simulink library "lib_joint_impctrl"  (Simulink 8.5)
settings: Solver=ode45  StartTime=0.0  StopTime=10.0  RelTol=1e-3
undefined symbols (not defined in the file): atlas_arm_lr, B, D, K_d, K_ext_c, K_ext_o, K_fri_o, K_O, K_obs_c, K_qD_d, K_qDD_d, K_tau_a, K_tau_c, K_tau_D, K_tau_e, K_tau_f, K_tau_g, K_tau_K, K_tau_o, MPV_arm_damp, MPV_arm_model, qD_th, T, T1, tau_c, tau_th
libraries: lib_joint_impctrl x7, atlas_dynamic_library x4
settings Model: Creator=knoechelmann  LastModifiedBy=prothese  CovSFcnEnable=off

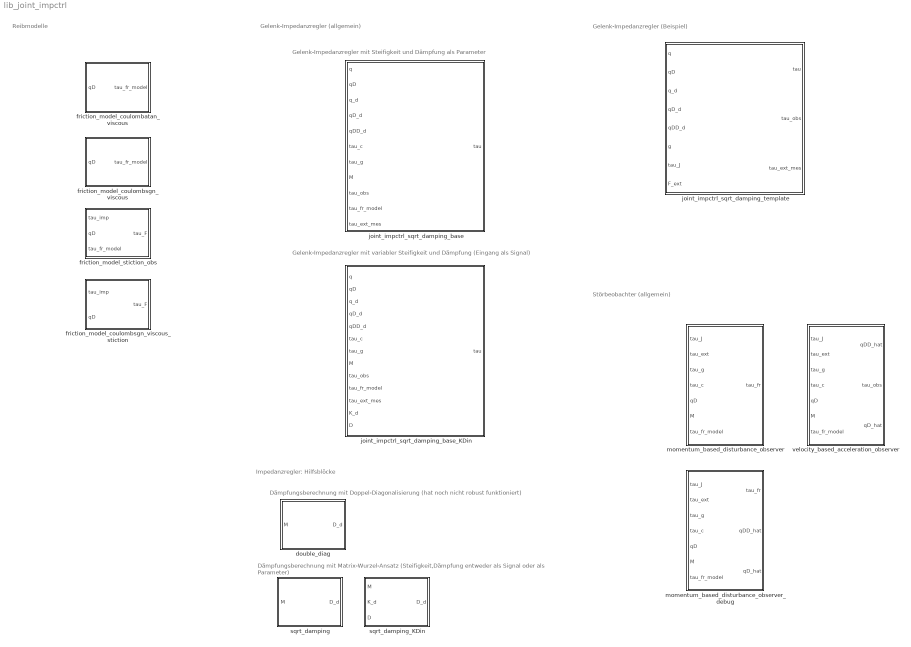
== system lib_joint_impctrl ==
  note: Dämpfungsberechnung mit Doppel-Diagonalisierung (hat noch nicht robust funktioniert)
  note: Dämpfungsberechnung mit Matrix-Wurzel-Ansatz (Steifigkeit,Dämpfung entweder als Signal oder als Parameter)
  note: Gelenk-Impedanzregler mit Steifigkeit und Dämpfung als Parameter
  note: Gelenk-Impedanzregler mit variabler Steifigkeit und Dämpfung (Eingang als Signal)
  note: Gelenk-Impedanzregler (Beispiel)
  note: Störbeobachter (allgemein)
  note: Gelenk-Impedanzregler (allgemein)
  note: Impedanzregler: Hilfsblöcke
  note: Reibmodelle
  double_diag : Subsystem  TreatAsAtomicUnit=on  mask{K_d=K_d, D=D}
  friction_model_coulombatan_viscous : Subsystem  TreatAsAtomicUnit=on  mask{tau_c=tau_c, B=B}
      mask prompts: tau_c "tau_c (vector with coulomb friction momentums for all joints)"; B "B (vector with viscous friction coefficients of all joints)"
  friction_model_coulombsgn_viscous : Subsystem  TreatAsAtomicUnit=on  mask{tau_c=tau_c, B=B}
      mask prompts: tau_c "tau_c (vector with coulomb friction momentums for all joints)"; B "B (vector with viscous friction coefficients of all joints)"
  friction_model_coulombsgn_viscous_stiction : Subsystem  TreatAsAtomicUnit=on  mask{tau_c=tau_c, B=B, qD_th=qD_th, tau_th=tau_th}
      mask prompts: tau_c "tau_c (vector with coulomb friction momentums for all joints)"; B "B (vector with viscous friction coefficients of all joints)"; qD_th "qD_th (vector with theshold velocities for stiction)"; tau_th "tau_th (vector with kick-in momentums for stiction compensation)"
  friction_model_stiction_obs : Subsystem  TreatAsAtomicUnit=on  mask{tau_c=tau_c, B=B, qD_th=qD_th, tau_th=tau_th}
      mask prompts: tau_c "tau_c (vector with coulomb friction momentums for all joints)"; B "B (vector with viscous friction coefficients of all joints)"; qD_th "qD_th (vector with theshold velocities for stiction)"; tau_th "tau_th (vector with kick-in momentums for stiction compensation)"
  joint_impctrl_sqrt_damping_base : Subsystem  TreatAsAtomicUnit=on  mask(Joint Impedance Controller Base){K_d=K_d, D=D, K_tau_g=K_tau_g, K_tau_c=K_tau_c, K_tau_K=K_tau_K, K_tau_D=K_tau_D, K_tau_a=K_tau_a, K_tau_f=K_tau_f, K_tau_e=K_tau_e, K_tau_o=K_tau_o, K_qD_d=K_qD_d, K_qDD_d=K_qDD_d, K_ext_c=K_ext_c, K_obs_c=K_obs_c, tau_c=tau_c, B=B, qD_th=qD_th, tau_th=tau_th}
      mask prompts: K_d "K_d (desired stiffness)"; D "D (diagonal matrix with desired damping coefficients)"; K_tau_g "K_tau_g (gain of gravity compensation)"; K_tau_c "K_tau_c (gain of corriolis- and inertia compensation)"; K_tau_K "K_tau_K (gain of stiffness component)"; K_tau_D "K_tau_D (gain of damping component)"; K_tau_a "K_tau_a (gain of acceleration component)"; K_tau_f "K_tau_f (gain of model based friction compensation)"; K_tau_e "K_tau_e (gain of compensation of external torque measurd via hand sensor)"; K_tau_o "K_tau_o (gain of compensation of disturbance observer torques)"; K_qD_d "K_qD_d (gain of desired velocity)"; K_qDD_d "K_qDD_d (gain of desired acceleration)"; K_ext_c "K_ext_c (input gain to deside, wether to trigger friction compensation via the measured external torque)"; K_obs_c "K_obs_c (input gain to deside, wether to trigger friction compensation via the observed torque)"; tau_c "tau_c (vector with coulomb friction momentums for all joints)"; B "B (vector with viscous friction coefficients of all joints)"; qD_th "qD_th (vector with theshold velocities for stiction)"; tau_th "tau_th (vector with kick-in momentums for stiction compensation)"
      mask help:
      | Hardware independent impedance controller base block with matrix
      | squareroot damping design. For a better testing, all partial mo-
      | mentums can be individually scaled. Coulomb-, viscous friction
      | and Stribeck stiction is taken into account for friction compen-
      | sation.
  joint_impctrl_sqrt_damping_base_KDin : Subsystem  TreatAsAtomicUnit=on  mask(Joint Impedance Controller Base){K_tau_g=K_tau_g, K_tau_c=K_tau_c, K_tau_K=K_tau_K, K_tau_D=K_tau_D, K_tau_a=K_tau_a, K_tau_f=K_tau_f, K_tau_e=K_tau_e, K_tau_o=K_tau_o, K_qD_d=K_qD_d, K_qDD_d=K_qDD_d, K_ext_c=K_ext_c, K_obs_c=K_obs_c, tau_c=tau_c, B=B, qD_th=qD_th, tau_th=tau_th}
      mask prompts: K_tau_g "K_tau_g (gain of gravity compensation)"; K_tau_c "K_tau_c (gain of corriolis- and inertia compensation)"; K_tau_K "K_tau_K (gain of stiffness component)"; K_tau_D "K_tau_D (gain of damping component)"; K_tau_a "K_tau_a (gain of acceleration component)"; K_tau_f "K_tau_f (gain of model based friction compensation)"; K_tau_e "K_tau_e (gain of compensation of external torque measurd via hand sensor)"; K_tau_o "K_tau_o (gain of compensation of disturbance observer torques)"; K_qD_d "K_qD_d (gain of desired velocity)"; K_qDD_d "K_qDD_d (gain of desired acceleration)"; K_ext_c "K_ext_c (input gain to deside, wether to trigger friction compensation via the measured external torque)"; K_obs_c "K_obs_c (input gain to deside, wether to trigger friction compensation via the observed torque)"; tau_c "tau_c (vector with coulomb friction momentums for all joints)"; B "B (vector with viscous friction coefficients of all joints)"; qD_th "qD_th (vector with theshold velocities for stiction)"; tau_th "tau_th (vector with kick-in momentums for stiction compensation)"
      mask help:
      | Hardware independent impedance controller base block with matrix
      | squareroot damping design. For a better testing, all partial mo-
      | mentums can be individually scaled. Coulomb-, viscous friction
      | and Stribeck stiction is taken into account for friction compen-
      | sation.
  joint_impctrl_sqrt_damping_template : Subsystem  TreatAsAtomicUnit=on  SystemSampleTime=T  mask(Atlas Joint Impedance Controller){K_d=K_d, D=D, K_tau_g=K_tau_g, K_tau_c=K_tau_c, K_tau_K=K_tau_K, K_tau_D=K_tau_D, K_tau_a=K_tau_a, K_tau_f=K_tau_f, K_tau_e=K_tau_e, K_tau_o=K_tau_o, K_qD_d=K_qD_d, K_qDD_d=K_qDD_d, K_ext_c=K_ext_c, K_obs_c=K_obs_c, K_fri_o=K_fri_o, K_ext_o=K_ext_o, MPV_arm_damp=MPV_arm_damp, MPV_arm_model=MPV_arm_model, tau_c=tau_c, B=B, qD_th=qD_th, tau_th=tau_th, K_O=K_O, T=T, atlas_arm_lr=atlas_arm_lr, T1=T1}
      mask prompts: K_d "K_d (desired stiffness)"; D "D (diagonal matrix with desired damping coefficients)"; K_tau_g "K_tau_g (gain of gravity compensation)"; K_tau_c "K_tau_c (gain of corriolis- and inertia compensation)"; K_tau_K "K_tau_K (gain of stiffness component)"; K_tau_D "K_tau_D (gain of damping component)"; K_tau_a "K_tau_a (gain of acceleration component)"; K_tau_f "K_tau_f (gain of model based friction compensation)"; K_tau_e "K_tau_e (gain of compensation of external torque measurd via hand sensor)"; K_tau_o "K_tau_o (gain of compensation of disturbance observer torques)"; K_qD_d "K_qD_d (gain of desired velocity)"; K_qDD_d "K_qDD_d (gain of desired acceleration)"; K_ext_c "K_ext_c (input gain to deside, wether to trigger friction compensation via the measured external torque)"; K_obs_c "K_obs_c (input gain to deside, wether to trigger friction compensation via the observed torque)"; K_fri_o "K_fri_o (input gain of friction model torques for observer)"; K_ext_o "K_ext_o (input gain of external torque for observer)"; MPV_arm_damp "MPV_damp (base parameter vector for damping calculation)"; MPV_arm_model "MPV_model (base parameter vector for dynamic model calculation)"; tau_c "tau_c (vector with coulomb friction momentums for all joints)"; B "B (vector with viscous friction coefficients of all joints)"; qD_th "qD_th (vector with theshold velocities for stiction)"; tau_th "tau_th (vector with kick-in momentums for stiction compensation)"; K_O "K_O (friction observer gain)"; T "T (sample time (important for friction observer))"; atlas_arm_lr "atlas_arm_lr (flag for left or right side)"; T1 "T1 (low pass filter time constant for inertia matrix)"
      mask help:
      | Hardware dependent full impedance controller block with matrix
      | squareroot damping design for the atlas robot. For a better
      | testing, all partial momentums can be individually scaled.
      | Coulomb-, viscous friction and Stribeck stiction is taken into
      | account for friction compensation.
  momentum_based_disturbance_observer : Subsystem  TreatAsAtomicUnit=on  SystemSampleTime=T  mask{K_O=K_O, T=T, T1=T1, tau_out_max=30*ones(6,1)}
      mask prompts: K_O "K_O (Observer gain)"; T "T (sampletime)"; T1 "T1 (low pass differentiator time constant)"; tau_out_max "tau_out_max (safety limit for output, output will be limited to lie in between -tau_out_max and tau_out_max)"
  momentum_based_disturbance_observer_debug : Subsystem  TreatAsAtomicUnit=on  SystemSampleTime=T  mask{K_O=K_O, T=T, T1=T1, tau_out_max=30*ones(6,1)}
      mask prompts: K_O "K_O (Observer gain)"; T "T (sampletime)"; T1 "T1 (low pass differentiator time constant)"; tau_out_max "tau_out_max (safety limit for output, output will be limited to lie in between -tau_out_max and tau_out_max)"
  sqrt_damping : Subsystem  TreatAsAtomicUnit=on  mask{K_d=K_d, D=D}
  sqrt_damping_KDin : Subsystem  TreatAsAtomicUnit=on
  velocity_based_acceleration_observer : Subsystem  TreatAsAtomicUnit=on  SystemSampleTime=T  mask{K_O=K_O, T=T}
      mask prompts: K_O "K_O (Observer gain)"; T "T (sampletime)"

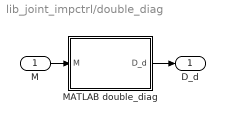
== system lib_joint_impctrl/double_diag ==
  M : Inport
  MATLAB double_diag : MATLAB Function  TreatAsAtomicUnit=on
  D_d : Outport
  wires:
  M/1 -> MATLAB double_diag/1(M)
  MATLAB double_diag/1(D_d) -> D_d/1

== system lib_joint_impctrl/friction_model_coulombatan_viscous ==
  qD : Inport
  atlas_friction_model_atan : MATLAB Function  TreatAsAtomicUnit=on
  tau_fr_model : Outport
  wires:
  qD/1 -> atlas_friction_model_atan/1(qD)
  atlas_friction_model_atan/1(tau_fr_model) -> tau_fr_model/1

== system lib_joint_impctrl/friction_model_coulombsgn_viscous ==
  qD : Inport
  atlas_friction_model : MATLAB Function  TreatAsAtomicUnit=on
  tau_fr_model : Outport
  wires:
  qD/1 -> atlas_friction_model/1(qD)
  atlas_friction_model/1(tau_fr_model) -> tau_fr_model/1

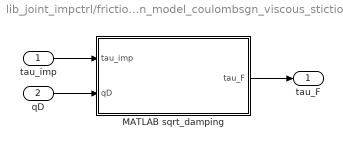
== system lib_joint_impctrl/friction_model_coulombsgn_viscous_stiction ==
  tau_imp : Inport
  qD : Inport  Port=2
  MATLAB sqrt_damping : MATLAB Function  TreatAsAtomicUnit=on
  tau_F : Outport
  wires:
  qD/1 -> MATLAB sqrt_damping/2(qD)
  MATLAB sqrt_damping/1(tau_F) -> tau_F/1
  tau_imp/1 -> MATLAB sqrt_damping/1(tau_imp)

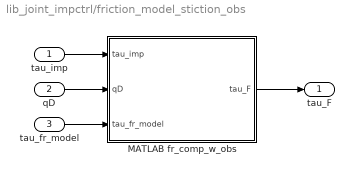
== system lib_joint_impctrl/friction_model_stiction_obs ==
  tau_imp : Inport
  qD : Inport  Port=2
  tau_fr_model : Inport  Port=3
  MATLAB fr_comp_w_obs : MATLAB Function  TreatAsAtomicUnit=on
  tau_F : Outport
  wires:
  qD/1 -> MATLAB fr_comp_w_obs/2(qD)
  MATLAB fr_comp_w_obs/1(tau_F) -> tau_F/1
  tau_imp/1 -> MATLAB fr_comp_w_obs/1(tau_imp)
  tau_fr_model/1 -> MATLAB fr_comp_w_obs/3(tau_fr_model)

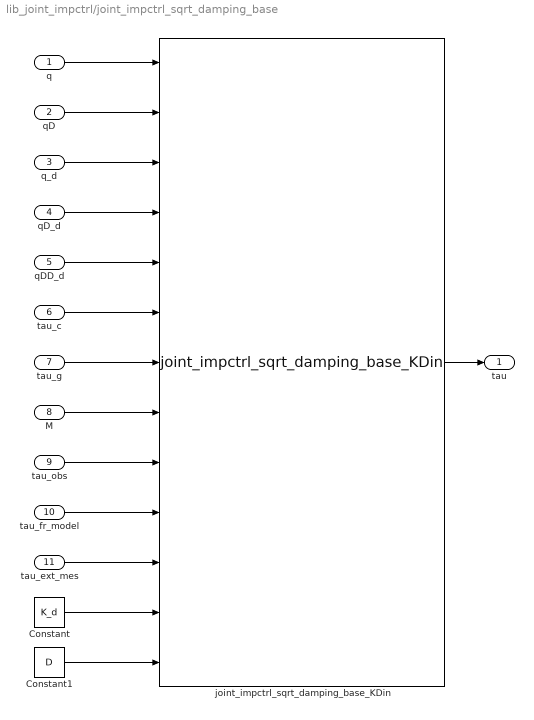
== system lib_joint_impctrl/joint_impctrl_sqrt_damping_base ==
  q : Inport
  qD : Inport  Port=2
  q_d : Inport  Port=3
  qD_d : Inport  Port=4
  qDD_d : Inport  Port=5
  tau_c : Inport  Port=6
  tau_g : Inport  Port=7
  M : Inport  Port=8
  tau_obs : Inport  Port=9
  tau_fr_model : Inport  Port=10
  tau_ext_mes : Inport  Port=11
  Constant : Constant  Value=K_d
  Constant1 : Constant  Value=D
  joint_impctrl_sqrt_damping_base_KDin : lib_joint_impctrl/joint_impctrl_sqrt_damping_base_KDin  K_tau_g=K_tau_g  K_tau_c=K_tau_c  K_tau_K=K_tau_K  K_tau_D=K_tau_D  K_tau_a=K_tau_a  K_tau_f=K_tau_f  K_tau_e=K_tau_e  K_tau_o=K_tau_o  K_qD_d=K_qD_d  K_qDD_d=K_qDD_d  K_ext_c=K_ext_c  K_obs_c=K_obs_c  tau_c=tau_c  B=B  qD_th=qD_th  tau_th=tau_th
  tau : Outport
  wires:
  joint_impctrl_sqrt_damping_base_KDin/1 -> tau/1
  tau_fr_model/1 -> joint_impctrl_sqrt_damping_base_KDin/10
  q/1 -> joint_impctrl_sqrt_damping_base_KDin/1
  q_d/1 -> joint_impctrl_sqrt_damping_base_KDin/3
  qD/1 -> joint_impctrl_sqrt_damping_base_KDin/2
  qD_d/1 -> joint_impctrl_sqrt_damping_base_KDin/4
  qDD_d/1 -> joint_impctrl_sqrt_damping_base_KDin/5
  tau_c/1 -> joint_impctrl_sqrt_damping_base_KDin/6
  tau_g/1 -> joint_impctrl_sqrt_damping_base_KDin/7
  tau_obs/1 -> joint_impctrl_sqrt_damping_base_KDin/9
  tau_ext_mes/1 -> joint_impctrl_sqrt_damping_base_KDin/11
  M/1 -> joint_impctrl_sqrt_damping_base_KDin/8
  Constant/1 -> joint_impctrl_sqrt_damping_base_KDin/12
  Constant1/1 -> joint_impctrl_sqrt_damping_base_KDin/13

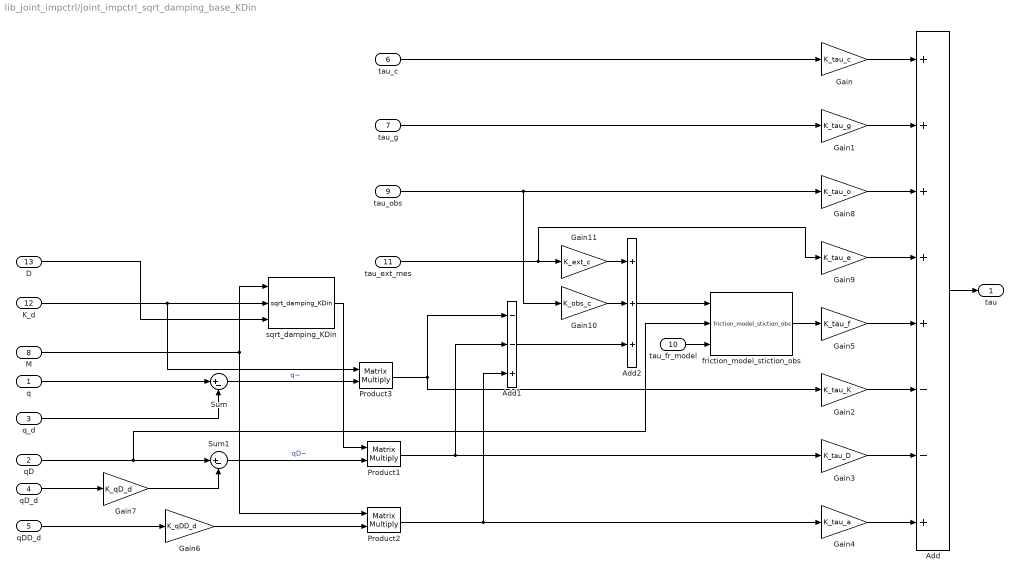
== system lib_joint_impctrl/joint_impctrl_sqrt_damping_base_KDin ==
  q : Inport
  qD : Inport  Port=2
  q_d : Inport  Port=3
  qD_d : Inport  Port=4
  qDD_d : Inport  Port=5
  tau_c : Inport  Port=6
  tau_g : Inport  Port=7
  M : Inport  Port=8
  tau_obs : Inport  Port=9
  tau_fr_model : Inport  Port=10
  tau_ext_mes : Inport  Port=11
  K_d : Inport  Port=12
  D : Inport  Port=13
  Add : Sum  Inputs=+++++--+
  Add1 : Sum  Inputs=--+
  Add2 : Sum  Inputs=+++
  Gain : Gain  Gain=K_tau_c
  Gain1 : Gain  Gain=K_tau_g
  Gain10 : Gain  Gain=K_obs_c
  Gain11 : Gain  Gain=K_ext_c
  Gain2 : Gain  Gain=K_tau_K
  Gain3 : Gain  Gain=K_tau_D
  Gain4 : Gain  Gain=K_tau_a
  Gain5 : Gain  Gain=K_tau_f
  Gain6 : Gain  Gain=K_qDD_d
  Gain7 : Gain  Gain=K_qD_d
  Gain8 : Gain  Gain=K_tau_o
  Gain9 : Gain  Gain=K_tau_e
  Product1 : Product  Multiplication=Matrix(*)
  Product2 : Product  Multiplication=Matrix(*)
  Product3 : Product  Multiplication=Matrix(*)
  Sum : Sum  Inputs=|+-
  Sum1 : Sum  Inputs=|+-
  friction_model_stiction_obs : lib_joint_impctrl/friction_model_stiction_obs  tau_c=tau_c  B=B  qD_th=qD_th  tau_th=tau_th
  sqrt_damping_KDin : lib_joint_impctrl/sqrt_damping_KDin  K_d=K_d  D=D
  tau : Outport
  wires:
  Gain6/1 -> Product2/2
  Gain7/1 -> Sum1/2
  q_d/1 -> Sum/2
  M/1 -> Product2/1, sqrt_damping_KDin/1
  q/1 -> Sum/1
  qD/1 -> friction_model_stiction_obs/2, Sum1/1
  qD_d/1 -> Gain7/1
  Sum1/1 -> Product1/2  "qD~"
  Sum/1 -> Product3/2  "q~"
  qDD_d/1 -> Gain6/1
  sqrt_damping_KDin/1 -> Product1/1
  Add/1 -> tau/1
  Product3/1 -> Gain2/1, Add1/1
  tau_g/1 -> Gain1/1
  tau_c/1 -> Gain/1
  Product1/1 -> Gain3/1, Add1/2
  Product2/1 -> Gain4/1, Add1/3
  Gain/1 -> Add/1
  Gain1/1 -> Add/2
  tau_obs/1 -> Gain8/1, Gain10/1
  tau_fr_model/1 -> friction_model_stiction_obs/3
  Gain5/1 -> Add/5
  Gain2/1 -> Add/6
  Gain3/1 -> Add/7
  Gain4/1 -> Add/8
  Gain8/1 -> Add/3
  tau_ext_mes/1 -> Gain9/1, Gain11/1
  Gain9/1 -> Add/4
  Add2/1 -> friction_model_stiction_obs/1
  Add1/1 -> Add2/3
  Gain10/1 -> Add2/2
  Gain11/1 -> Add2/1
  friction_model_stiction_obs/1 -> Gain5/1
  K_d/1 -> Product3/1, sqrt_damping_KDin/2
  D/1 -> sqrt_damping_KDin/3

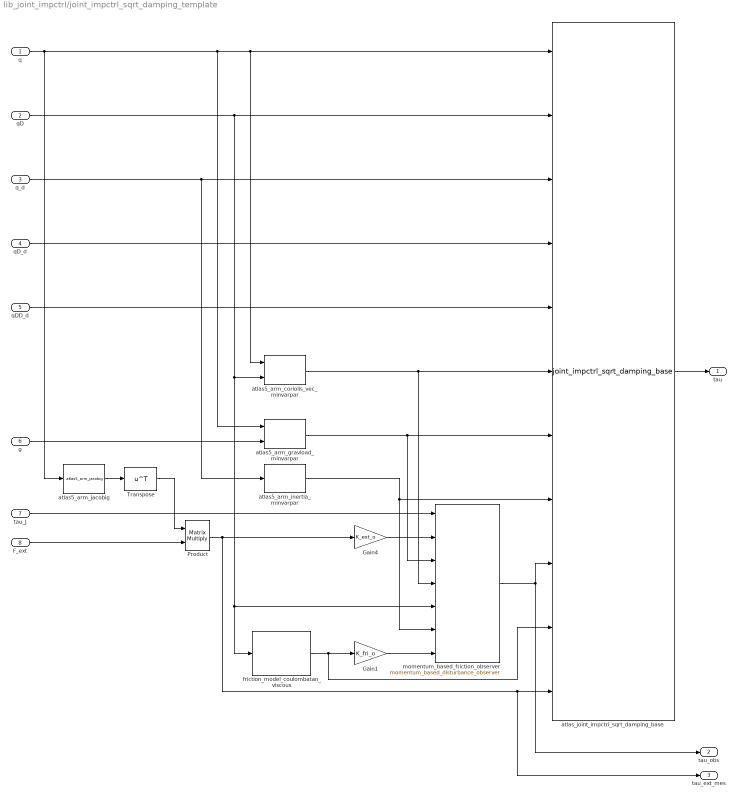
== system lib_joint_impctrl/joint_impctrl_sqrt_damping_template ==
  q : Inport  OutDataTypeStr=double  PortDimensions=7
  qD : Inport  Port=2  OutDataTypeStr=double  PortDimensions=7
  q_d : Inport  Port=3  OutDataTypeStr=double  PortDimensions=7
  qD_d : Inport  Port=4  OutDataTypeStr=double  PortDimensions=7
  qDD_d : Inport  Port=5  OutDataTypeStr=double  PortDimensions=7
  g : Inport  Port=6  OutDataTypeStr=double  PortDimensions=3
  tau_J : Inport  Port=7  OutDataTypeStr=double  PortDimensions=7
  F_ext : Inport  Port=8  OutDataTypeStr=double  PortDimensions=6
  Gain1 : Gain  Gain=K_fri_o
  Gain4 : Gain  Gain=K_ext_o
  Product : Product  Multiplication=Matrix(*)
  Transpose : Math  Operator=transpose  SaturateOnIntegerOverflow=on
  atlas5_arm_coriolis_vec_minvarpar : atlas_dynamic_library/atlas5_arm_coriolis_vec_minvarpar  atlas_arm_lr=atlas_arm_lr  MPV=MPV_arm_model
  atlas5_arm_gravload_minvarpar : atlas_dynamic_library/atlas5_arm_gravload_minvarpar  atlas_arm_lr=atlas_arm_lr  MPV=MPV_arm_model
  atlas5_arm_inertia_minvarpar : atlas_dynamic_library/atlas5_arm_inertia_minvarpar  atlas_arm_lr=atlas_arm_lr  MPV=MPV_arm_damp
  atlas5_arm_jacobig : atlas_dynamic_library/atlas5_arm_jacobig
  atlas_joint_impctrl_sqrt_damping_base : lib_joint_impctrl/joint_impctrl_sqrt_damping_base  K_d=K_d  D=D  K_tau_g=K_tau_g  K_tau_c=K_tau_c  K_tau_K=K_tau_K  K_tau_D=K_tau_D  K_tau_a=K_tau_a  K_tau_f=K_tau_f  K_tau_e=K_tau_e  K_tau_o=K_tau_o  K_qD_d=K_qD_d  K_qDD_d=K_qDD_d  K_ext_c=K_ext_c  K_obs_c=K_obs_c  tau_c=tau_c  B=B  qD_th=qD_th  tau_th=tau_th
  friction_model_coulombatan_viscous : lib_joint_impctrl/friction_model_coulombatan_viscous  tau_c=tau_c  B=B
  momentum_based_friction_observer : lib_joint_impctrl/momentum_based_disturbance_observer  K_O=K_O  T=T  T1=T1  tau_out_max=30*ones(7,1)
  tau : Outport  OutDataTypeStr=double  PortDimensions=7
  tau_obs : Outport  Port=2  OutDataTypeStr=double  PortDimensions=7
  tau_ext_mes : Outport  Port=3  OutDataTypeStr=double  PortDimensions=7
  wires:
  atlas_joint_impctrl_sqrt_damping_base/1 -> tau/1
  atlas5_arm_inertia_minvarpar/1 -> momentum_based_friction_observer/6, atlas_joint_impctrl_sqrt_damping_base/8
  q/1 -> atlas5_arm_jacobig/1, atlas5_arm_gravload_minvarpar/1, atlas5_arm_coriolis_vec_minvarpar/1, atlas_joint_impctrl_sqrt_damping_base/1
  qD/1 -> atlas_joint_impctrl_sqrt_damping_base/2, atlas5_arm_coriolis_vec_minvarpar/2, friction_model_coulombatan_viscous/1, momentum_based_friction_observer/5
  q_d/1 -> atlas5_arm_inertia_minvarpar/1, atlas_joint_impctrl_sqrt_damping_base/3
  atlas5_arm_coriolis_vec_minvarpar/1 -> momentum_based_friction_observer/4, atlas_joint_impctrl_sqrt_damping_base/6
  qD_d/1 -> atlas_joint_impctrl_sqrt_damping_base/4
  atlas5_arm_gravload_minvarpar/1 -> momentum_based_friction_observer/3, atlas_joint_impctrl_sqrt_damping_base/7
  qDD_d/1 -> atlas_joint_impctrl_sqrt_damping_base/5
  g/1 -> atlas5_arm_gravload_minvarpar/2
  momentum_based_friction_observer/1 -> tau_obs/1, atlas_joint_impctrl_sqrt_damping_base/9
  tau_J/1 -> momentum_based_friction_observer/1
  atlas5_arm_jacobig/1 -> Transpose/1
  Transpose/1 -> Product/1
  F_ext/1 -> Product/2
  Product/1 -> tau_ext_mes/1, atlas_joint_impctrl_sqrt_damping_base/11, Gain4/1
  friction_model_coulombatan_viscous/1 -> atlas_joint_impctrl_sqrt_damping_base/10, Gain1/1
  Gain4/1 -> momentum_based_friction_observer/2
  Gain1/1 -> momentum_based_friction_observer/7

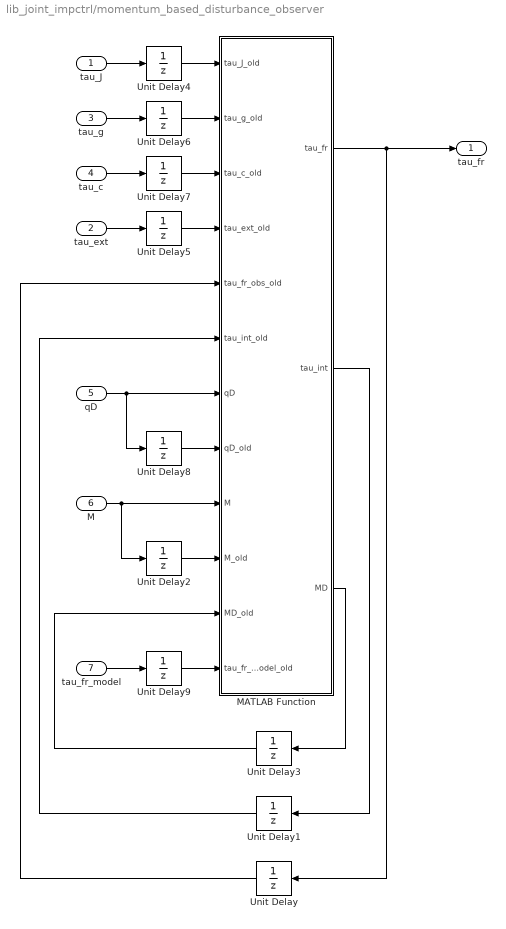
== system lib_joint_impctrl/momentum_based_disturbance_observer ==
  tau_J : Inport  OutDataTypeStr=double
  tau_ext : Inport  Port=2  OutDataTypeStr=double
  tau_g : Inport  Port=3  OutDataTypeStr=double
  tau_c : Inport  Port=4  OutDataTypeStr=double
  qD : Inport  Port=5  OutDataTypeStr=double
  M : Inport  Port=6  OutDataTypeStr=double
  tau_fr_model : Inport  Port=7  OutDataTypeStr=double
  MATLAB Function : MATLAB Function  TreatAsAtomicUnit=on
  Unit Delay{,1..9} (10 alike) : UnitDelay  SampleTime=-1
  tau_fr : Outport  OutDataTypeStr=double
  wires:
  Unit Delay/1 -> MATLAB Function/5(tau_fr_obs_old)
  tau_g/1 -> Unit Delay6/1
  tau_J/1 -> Unit Delay4/1
  M/1 -> Unit Delay2/1, MATLAB Function/9(M)
  qD/1 -> Unit Delay8/1, MATLAB Function/7(qD)
  tau_c/1 -> Unit Delay7/1
  MATLAB Function/2(tau_int) -> Unit Delay1/1
  Unit Delay1/1 -> MATLAB Function/6(tau_int_old)
  Unit Delay2/1 -> MATLAB Function/10(M_old)
  MATLAB Function/3(MD) -> Unit Delay3/1
  Unit Delay3/1 -> MATLAB Function/11(MD_old)
  Unit Delay4/1 -> MATLAB Function/1(tau_J_old)
  Unit Delay6/1 -> MATLAB Function/2(tau_g_old)
  Unit Delay7/1 -> MATLAB Function/3(tau_c_old)
  Unit Delay8/1 -> MATLAB Function/8(qD_old)
  MATLAB Function/1(tau_fr) -> Unit Delay/1, tau_fr/1
  tau_ext/1 -> Unit Delay5/1
  Unit Delay5/1 -> MATLAB Function/4(tau_ext_old)
  tau_fr_model/1 -> Unit Delay9/1
  Unit Delay9/1 -> MATLAB Function/12(tau_fr_model_old)

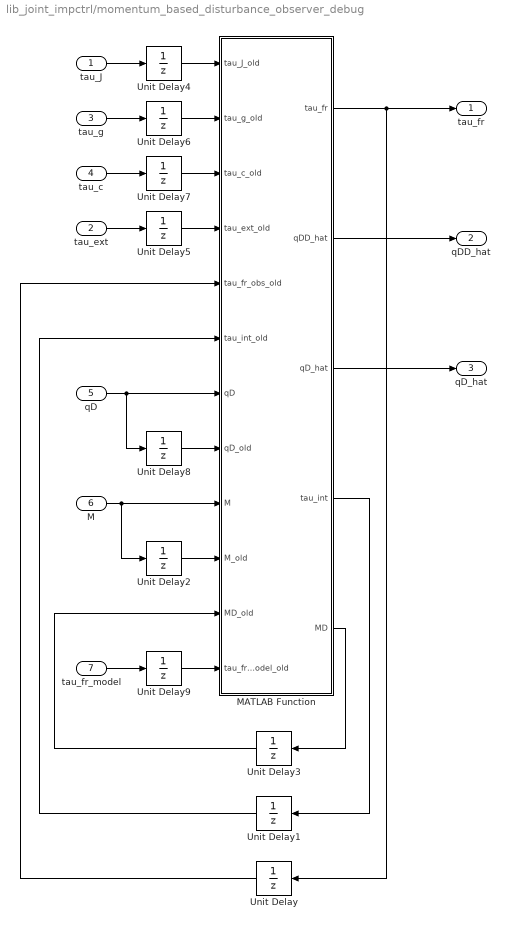
== system lib_joint_impctrl/momentum_based_disturbance_observer_debug ==
  tau_J : Inport  OutDataTypeStr=double
  tau_ext : Inport  Port=2  OutDataTypeStr=double
  tau_g : Inport  Port=3  OutDataTypeStr=double
  tau_c : Inport  Port=4  OutDataTypeStr=double
  qD : Inport  Port=5  OutDataTypeStr=double
  M : Inport  Port=6  OutDataTypeStr=double
  tau_fr_model : Inport  Port=7  OutDataTypeStr=double
  MATLAB Function : MATLAB Function  TreatAsAtomicUnit=on
  Unit Delay{,1..9} (10 alike) : UnitDelay  SampleTime=-1
  tau_fr : Outport  OutDataTypeStr=double
  qDD_hat : Outport  Port=2  OutDataTypeStr=double
  qD_hat : Outport  Port=3  OutDataTypeStr=double
  wires:
  Unit Delay/1 -> MATLAB Function/5(tau_fr_obs_old)
  tau_g/1 -> Unit Delay6/1
  tau_J/1 -> Unit Delay4/1
  M/1 -> Unit Delay2/1, MATLAB Function/9(M)
  qD/1 -> Unit Delay8/1, MATLAB Function/7(qD)
  tau_c/1 -> Unit Delay7/1
  MATLAB Function/4(tau_int) -> Unit Delay1/1
  Unit Delay1/1 -> MATLAB Function/6(tau_int_old)
  Unit Delay2/1 -> MATLAB Function/10(M_old)
  MATLAB Function/5(MD) -> Unit Delay3/1
  Unit Delay3/1 -> MATLAB Function/11(MD_old)
  Unit Delay4/1 -> MATLAB Function/1(tau_J_old)
  Unit Delay6/1 -> MATLAB Function/2(tau_g_old)
  Unit Delay7/1 -> MATLAB Function/3(tau_c_old)
  Unit Delay8/1 -> MATLAB Function/8(qD_old)
  MATLAB Function/1(tau_fr) -> Unit Delay/1, tau_fr/1
  tau_ext/1 -> Unit Delay5/1
  Unit Delay5/1 -> MATLAB Function/4(tau_ext_old)
  tau_fr_model/1 -> Unit Delay9/1
  Unit Delay9/1 -> MATLAB Function/12(tau_fr_model_old)
  MATLAB Function/2(qDD_hat) -> qDD_hat/1
  MATLAB Function/3(qD_hat) -> qD_hat/1

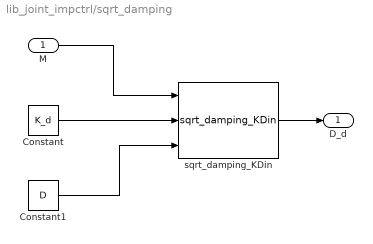
== system lib_joint_impctrl/sqrt_damping ==
  M : Inport
  Constant : Constant  Value=K_d
  Constant1 : Constant  Value=D
  sqrt_damping_KDin : lib_joint_impctrl/sqrt_damping_KDin  K_d=K_d  D=D
  D_d : Outport
  wires:
  M/1 -> sqrt_damping_KDin/1
  sqrt_damping_KDin/1 -> D_d/1
  Constant/1 -> sqrt_damping_KDin/2
  Constant1/1 -> sqrt_damping_KDin/3

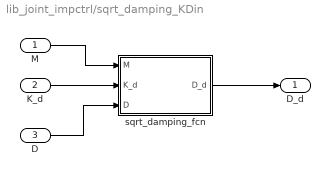
== system lib_joint_impctrl/sqrt_damping_KDin ==
  M : Inport
  K_d : Inport  Port=2
  D : Inport  Port=3
  sqrt_damping_fcn : MATLAB Function  TreatAsAtomicUnit=on
  D_d : Outport
  wires:
  M/1 -> sqrt_damping_fcn/1(M)
  sqrt_damping_fcn/1(D_d) -> D_d/1
  K_d/1 -> sqrt_damping_fcn/2(K_d)
  D/1 -> sqrt_damping_fcn/3(D)

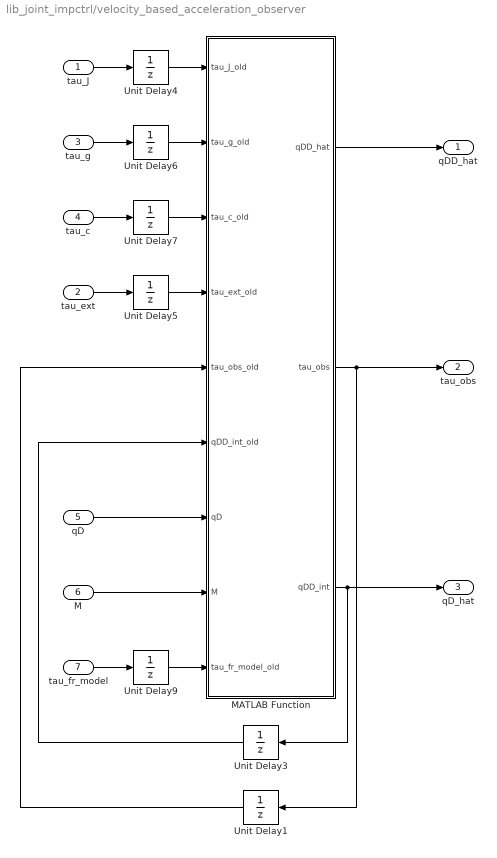
== system lib_joint_impctrl/velocity_based_acceleration_observer ==
  tau_J : Inport  OutDataTypeStr=double
  tau_ext : Inport  Port=2  OutDataTypeStr=double
  tau_g : Inport  Port=3  OutDataTypeStr=double
  tau_c : Inport  Port=4  OutDataTypeStr=double
  qD : Inport  Port=5  OutDataTypeStr=double
  M : Inport  Port=6  OutDataTypeStr=double
  tau_fr_model : Inport  Port=7  OutDataTypeStr=double
  MATLAB Function : MATLAB Function  TreatAsAtomicUnit=on
  Unit Delay{1,3..7,9} (7 alike) : UnitDelay  SampleTime=-1
  qDD_hat : Outport  OutDataTypeStr=double
  tau_obs : Outport  Port=2  OutDataTypeStr=double
  qD_hat : Outport  Port=3  OutDataTypeStr=double
  wires:
  tau_g/1 -> Unit Delay6/1
  tau_J/1 -> Unit Delay4/1
  M/1 -> MATLAB Function/8(M)
  qD/1 -> MATLAB Function/7(qD)
  tau_c/1 -> Unit Delay7/1
  MATLAB Function/2(tau_obs) -> tau_obs/1, Unit Delay1/1
  MATLAB Function/3(qDD_int) -> Unit Delay3/1, qD_hat/1
  Unit Delay4/1 -> MATLAB Function/1(tau_J_old)
  Unit Delay6/1 -> MATLAB Function/2(tau_g_old)
  Unit Delay7/1 -> MATLAB Function/3(tau_c_old)
  MATLAB Function/1(qDD_hat) -> qDD_hat/1
  tau_ext/1 -> Unit Delay5/1
  Unit Delay5/1 -> MATLAB Function/4(tau_ext_old)
  tau_fr_model/1 -> Unit Delay9/1
  Unit Delay9/1 -> MATLAB Function/9(tau_fr_model_old)
  Unit Delay3/1 -> MATLAB Function/6(qDD_int_old)
  Unit Delay1/1 -> MATLAB Function/5(tau_obs_old)

== matlab function double_diag/MATLAB double_diag ==
  data: M input double; K_d parameter double; D_d output double; D parameter double
function D_d=double_diag(M,K_d,D)
%#codegen
[V,K0]=eig(K_d,M);
% Q=inv(V)';
% D_d_=2*Q*D*sqrt(K0)*Q';
QD=V'\D;
Y=2*QD*sqrt(K0);
D_d_=Y/V;
assert(max(max(abs(imag(D_d_))))==0);
D_d=real(D_d_);

== matlab function velocity_based_acceleration_observer/MATLAB Function ==
  data: tau_J_old input double; qDD_hat output double; tau_g_old input double; tau_c_old input double; tau_ext_old input double; tau_obs_old input double; qDD_int_old input double; qD input double; M input double; tau_fr_model_old input double; K_O parameter double; T parameter double size=[1 1]; tau_obs output double; qDD_int output double
function [qDD_hat, tau_obs, qDD_int] = fcn(tau_J_old, tau_g_old, tau_c_old, tau_ext_old, tau_obs_old, qDD_int_old, qD, M, tau_fr_model_old, K_O, T)
%#codegen

qDD_hat = M\(tau_J_old-tau_g_old-tau_c_old+tau_obs_old+tau_ext_old-tau_fr_model_old);
qDD_int = qDD_int_old + T*qDD_hat;
tau_obs = K_O*(qD - qDD_int);

== matlab function momentum_based_disturbance_observer_debug/MATLAB Function ==
  data: tau_J_old input double; tau_fr output double; qDD_hat output double; qD_hat output double; tau_g_old input double; tau_c_old input double; tau_ext_old input double; tau_fr_obs_old input double; tau_int_old input double; qD input double; qD_old input double; M input double; M_old input double; MD_old input double; tau_fr_model_old input double; K_O parameter double; T1 parameter double size=[1 1]; tau_out_max parameter double; T parameter double size=[1 1]; tau_int output double; MD output double
function [tau_fr, qDD_hat, qD_hat, tau_int, MD] = fcn(tau_J_old, tau_g_old, tau_c_old, tau_ext_old, tau_fr_obs_old, tau_int_old, qD, qD_old, M, M_old, MD_old, tau_fr_model_old, K_O, T1, tau_out_max, T)
%#codegen

MD      = 1/(T1+T) * (T1*MD_old + M - M_old);
pD_hat = tau_J_old-tau_g_old-tau_c_old+MD*qD_old+tau_fr_obs_old+tau_ext_old-tau_fr_model_old;
qDD_hat = M\(pD_hat-MD*qD_old);
tau_int = tau_int_old + T*pD_hat;
qD_hat = M\tau_int;
tau_fr_MqD = K_O*(M*qD);
tau_fr = tau_fr_MqD - K_O*tau_int;

% limit output and anti-windup
for i=1:length(tau_J_old)
  if tau_fr(i)>tau_out_max(i)
    tau_fr(i)=tau_out_max(i);
    tau_int(i)=1/K_O(i,i)*(tau_fr_MqD(i)-tau_out_max(i));
  elseif tau_fr(i)<-tau_out_max(i)
    tau_fr(i)=-tau_out_max(i);
    tau_int(i)=1/K_O(i,i)*(tau_fr_MqD(i)+tau_out_max(i));
  end
end

== matlab function sqrt_damping_KDin/sqrt_damping_fcn ==
  data: M input double; K_d input double; D_d output double; D input double
function D_d=sqrt_damping(M,K_d,D)
%#codegen
K_d1=sqrtm(K_d);
M1=sqrtm(M);
D_d_=K_d1*D*M1+M1*D*K_d1;
assert(max(max(abs(imag(D_d_))))==0, ...
  'sqrt_damping: Damping Matrix has imaginary parts');
D_d=real(D_d_);

== matlab function friction_model_coulombsgn_viscous_stiction/MATLAB sqrt_damping ==
  data: tau_imp input double; qD input double; tau_F output double; tau_c parameter double; B parameter double; qD_th parameter double; tau_th parameter double
function tau_F=sqrt_damping(tau_imp,qD,tau_c,B,qD_th,tau_th)
%#codegen
tau_F=zeros(length(tau_imp),1);
for i=1:length(tau_imp)
  % friction compensation only, when significant distance to desired
  % trajectory
  if (abs(tau_imp(i)) > tau_th(i))
    % when qD<qD_th stiction is assumed and even if speed is in opposite
    % direction, full compensation force is applied, this is to avoid
    % sensor noise induced jitter
    if (abs(qD(i)) > qD_th(i) || sign(qD(i))==sign(tau_imp(i)))
      tau_F(i) = tau_c(i)*sign(qD(i)) + B(i)*qD(i);
    else
      tau_F(i) = tau_c(i);
    end
  else
    tau_F(i) = 0;
  end
end

== matlab function momentum_based_disturbance_observer/MATLAB Function ==
  data: tau_J_old input double; tau_fr output double; tau_g_old input double; tau_c_old input double; tau_ext_old input double; tau_fr_obs_old input double; tau_int_old input double; qD input double; qD_old input double; M input double; M_old input double; MD_old input double; tau_fr_model_old input double; K_O parameter double; T1 parameter double size=[1 1]; tau_out_max parameter double; T parameter double size=[1 1]; tau_int output double; MD output double
function [tau_fr, tau_int, MD] = fcn(tau_J_old, tau_g_old, tau_c_old, tau_ext_old, tau_fr_obs_old, tau_int_old, qD, qD_old, M, M_old, MD_old, tau_fr_model_old, K_O, T1, tau_out_max, T)
%#codegen

MD      = 1/(T1+T) * (T1*MD_old + M - M_old);
tau_int = tau_int_old + T*(tau_J_old-tau_g_old-tau_c_old+MD*qD_old+tau_fr_obs_old+tau_ext_old-tau_fr_model_old);
tau_fr_MqD = K_O*(M*qD);
tau_fr = tau_fr_MqD - K_O*tau_int;

% limit output and anti-windup
for i=1:length(tau_J_old)
  if tau_fr(i)>tau_out_max(i)
    tau_fr(i)=tau_out_max(i);
    tau_int(i)=1/K_O(i,i)*(tau_fr_MqD(i)-tau_out_max(i));
  elseif tau_fr(i)<-tau_out_max(i)
    tau_fr(i)=-tau_out_max(i);
    tau_int(i)=1/K_O(i,i)*(tau_fr_MqD(i)+tau_out_max(i));
  end
end

== matlab function friction_model_stiction_obs/MATLAB fr_comp_w_obs ==
  data: tau_imp input double; qD input double; tau_F output double; tau_fr_model input double; tau_c parameter double; qD_th parameter double; tau_th parameter double
function tau_F=fr_comp_w_obs(tau_imp,qD,tau_fr_model,tau_c,qD_th,tau_th)
%#codegen
tau_F=zeros(length(tau_imp),1);
for i=1:length(tau_imp)
  if (abs(qD(i)) > qD_th(i))
    tau_F(i) = tau_fr_model(i);
  else
    % for low speed friction compensation only, when significant distance
    % to desired trajectory
    if (abs(tau_imp(i)) > tau_th(i))
      % when qD<qD_th stiction is assumed and even if speed is in opposite
      % direction, full compensation force is applied, this is to avoid
      % sensor noise induced jitter
      if (sign(qD(i))==sign(tau_imp(i)))
        tau_F(i) = tau_fr_model(i);
      else
        tau_F(i) = tau_c(i);
      end
    else
      tau_F(i) = 0;
    end
  end
end

== matlab function friction_model_coulombatan_viscous/atlas_friction_model_atan ==
  data: qD input double; tau_fr_model output double; tau_c parameter double; B parameter double
function tau_fr_model = fcn(qD, tau_c, B)
%#codegen
tau_fr_model=zeros(length(qD),1);
for i=1:length(qD)
  tau_fr_model(i)=tau_c(i)*2/pi*atan(100*qD(i)) + B(i)*qD(i);
end

== matlab function friction_model_coulombsgn_viscous/atlas_friction_model ==
  data: qD input double; tau_fr_model output double; tau_c parameter double; B parameter double
function tau_fr_model = fcn(qD, tau_c, B)
%#codegen
tau_fr_model=zeros(length(qD),1);
for i=1:length(qD)
  tau_fr_model(i)=tau_c(i)*sign(qD(i)) + B(i)*qD(i);
end
